simulink model "simulink_model_project"  (R2022b)
settings: Solver=VariableStepAuto  StartTime=0.0  StopTime=10  RelTol=1e-3
values from neighbouring files (symbols this model uses):
  A = [0, 1, 0, 0; -k1/m1, -b1/m1, k1/m1, b1/m1; 0, 0, 0, 1; k1/m2, b1/m2, -(k1 + k2)/m2, -(b1 + b2)/m2]    [project_code_main.m]
  B = [0, 0; 0, 0; 0, 0; k2/m2, b2/m2]    [project_code_main.m]
  C = [1, 0, 0, 0; 0, 0, 1, 0]    [project_code_main.m]
  D = [0, 0; 0, 0]    [project_code_main.m]
settings Model: Creator=zafee  LastModifiedBy=zafee

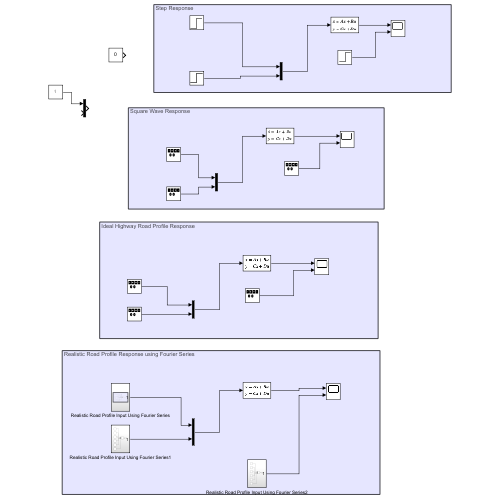
[thumbnail: Simulink's stored preview of the top-level diagram]
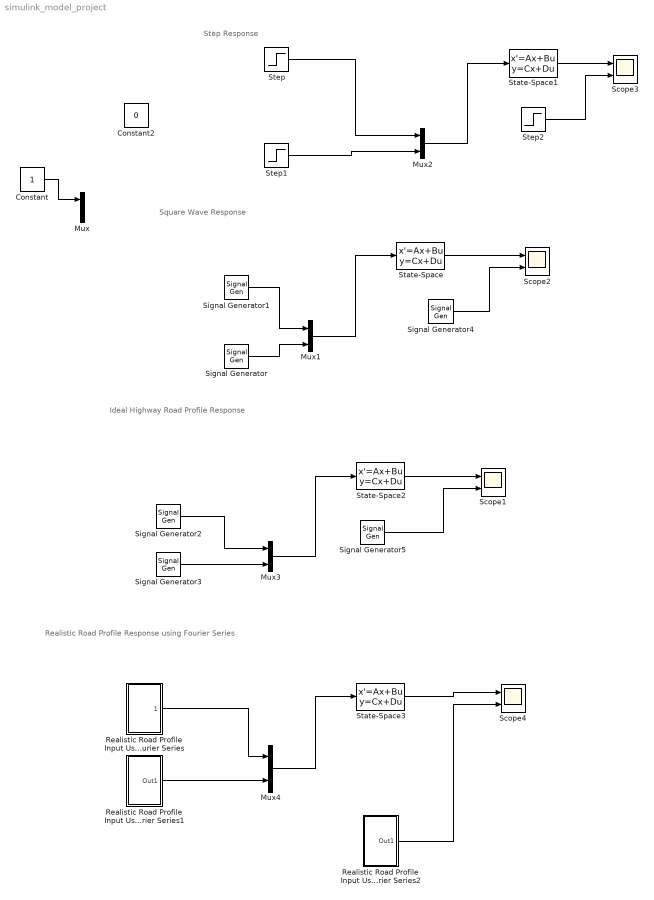
== system simulink_model_project ==
  note: Realistic Road Profile Response using Fourier Series
  note: Ideal Highway Road Profile Response
  note: Step Response
  note: Square Wave Response
  Constant : Constant
  Constant2 : Constant  Value=0
  Mux{,1..4} (5 alike) : Mux  Inputs=2
  Realistic Road Profile Input Using Fourier Series : Subsystem
  Realistic Road Profile Input Using Fourier Series1 : Subsystem
  Realistic Road Profile Input Using Fourier Series2 : Subsystem
  Scope{1..4} (4 alike) : Scope  NumInputPorts=2
  Signal Generator : SignalGenerator  WaveForm=square  Amplitude=0.1  Frequency=0.2
  Signal Generator1 : SignalGenerator  WaveForm=square  Amplitude=0.1  Frequency=0.2
  Signal Generator2 : SignalGenerator  Amplitude=0.015  Frequency=17.28513944  Units=rad/sec
  Signal Generator3 : SignalGenerator  Amplitude=0.015  Frequency=17.28513944  Units=rad/sec
  Signal Generator4 : SignalGenerator  WaveForm=square  Amplitude=0.1  Frequency=0.2
  Signal Generator5 : SignalGenerator  Amplitude=0.015  Frequency=17.28513944  Units=rad/sec
  State-Space{,1..3} (4 alike) : StateSpace  A=A  B=B  C=C  D=D  InitialCondition=0
  Step : Step  Time=0  After=0.1  SampleTime=0
  Step1 : Step  Time=0  After=0.1  SampleTime=0
  Step2 : Step  Time=0  After=0.1  SampleTime=0
  wires:
  Step/1 -> Mux2/1
  Step1/1 -> Mux2/2
  Constant/1 -> Mux/1
  Mux1/1 -> State-Space/1
  Signal Generator/1 -> Mux1/2
  Signal Generator1/1 -> Mux1/1
  Mux2/1 -> State-Space1/1
  Mux3/1 -> State-Space2/1
  Signal Generator3/1 -> Mux3/2
  Signal Generator2/1 -> Mux3/1
  State-Space3/1 -> Scope4/1
  Mux4/1 -> State-Space3/1
  Realistic Road Profile Input Using Fourier Series1/1(Out1) -> Mux4/2
  Realistic Road Profile Input Using Fourier Series/1(Output) -> Mux4/1
  Realistic Road Profile Input Using Fourier Series2/1(Out1) -> Scope4/2
  State-Space1/1 -> Scope3/1
  State-Space/1 -> Scope2/1
  State-Space2/1 -> Scope1/1
  Step2/1 -> Scope3/2
  Signal Generator4/1 -> Scope2/2
  Signal Generator5/1 -> Scope1/2

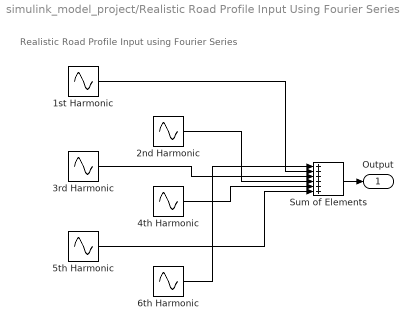
== system simulink_model_project/Realistic Road Profile Input Using Fourier Series ==
  note: Realistic Road Profile Input using Fourier Series
  1st Harmonic : Sin  Amplitude=0.01  SampleTime=0
  2nd Harmonic : Sin  Amplitude=0.01  Frequency=2  SampleTime=0
  3rd Harmonic : Sin  Amplitude=0.002  Frequency=3  SampleTime=0
  4th Harmonic : Sin  Amplitude=0.001  Frequency=4  SampleTime=0
  5th Harmonic : Sin  Amplitude=0.001  Frequency=5  SampleTime=0
  6th Harmonic : Sin  Amplitude=0.002  Frequency=6  SampleTime=0
  Sum of Elements : Sum  Inputs=++++++
  Output : Outport
  wires:
  3rd Harmonic/1 -> Sum of Elements/3
  4th Harmonic/1 -> Sum of Elements/5
  2nd Harmonic/1 -> Sum of Elements/4
  1st Harmonic/1 -> Sum of Elements/2
  5th Harmonic/1 -> Sum of Elements/6
  Sum of Elements/1 -> Output/1
  6th Harmonic/1 -> Sum of Elements/1

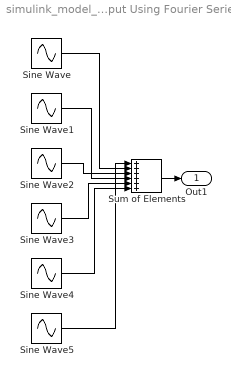
== system simulink_model_project/Realistic Road Profile Input Using Fourier Series1 ==
  Sine Wave : Sin  Amplitude=0.01  SampleTime=0
  Sine Wave1 : Sin  Amplitude=0.01  Frequency=2  SampleTime=0
  Sine Wave2 : Sin  Amplitude=0.002  Frequency=3  SampleTime=0
  Sine Wave3 : Sin  Amplitude=0.001  Frequency=4  SampleTime=0
  Sine Wave4 : Sin  Amplitude=0.001  Frequency=5  SampleTime=0
  Sine Wave5 : Sin  Amplitude=0.002  Frequency=6  SampleTime=0
  Sum of Elements : Sum  Inputs=++++++
  Out1 : Outport
  wires:
  Sine Wave5/1 -> Sum of Elements/1
  Sum of Elements/1 -> Out1/1
  Sine Wave4/1 -> Sum of Elements/6
  Sine Wave/1 -> Sum of Elements/2
  Sine Wave1/1 -> Sum of Elements/4
  Sine Wave3/1 -> Sum of Elements/5
  Sine Wave2/1 -> Sum of Elements/3

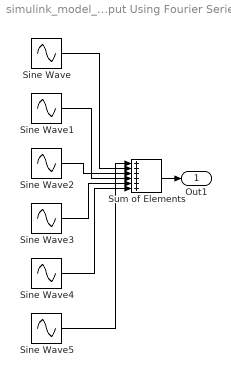
== system simulink_model_project/Realistic Road Profile Input Using Fourier Series2 ==
  Sine Wave : Sin  Amplitude=0.01  SampleTime=0
  Sine Wave1 : Sin  Amplitude=0.01  Frequency=2  SampleTime=0
  Sine Wave2 : Sin  Amplitude=0.002  Frequency=3  SampleTime=0
  Sine Wave3 : Sin  Amplitude=0.001  Frequency=4  SampleTime=0
  Sine Wave4 : Sin  Amplitude=0.001  Frequency=5  SampleTime=0
  Sine Wave5 : Sin  Amplitude=0.002  Frequency=6  SampleTime=0
  Sum of Elements : Sum  Inputs=++++++
  Out1 : Outport
  wires:
  Sine Wave5/1 -> Sum of Elements/1
  Sum of Elements/1 -> Out1/1
  Sine Wave4/1 -> Sum of Elements/6
  Sine Wave/1 -> Sum of Elements/2
  Sine Wave1/1 -> Sum of Elements/4
  Sine Wave3/1 -> Sum of Elements/5
  Sine Wave2/1 -> Sum of Elements/3
